simulink model "simu_v3"  (R2021a)
settings: Solver=VariableStepAuto  StartTime=0.0  StopTime=200  RelTol=1e-3
model workspace: external: MATLAB File G:\My Drive\0. PUCP\Cursos\2020.2\IEE243 - Sistemas de Control\Tarea Academica\Simulacion Robot Movil\cad files\RobotMovil_DataFile.m (data not in the file)
values from neighbouring files (symbols this model uses):
  xPla = 3    [RobotMovil_DataFile.m]
  yPla = 3    [RobotMovil_DataFile.m]
  zPla = 0.001    [RobotMovil_DataFile.m]
undefined symbols (not defined in the file or in its folder): smiData, X, Y, Z
libraries: sm_lib x211, nesl_utility x6, simulink x3, fl_lib x3
(part 5 of 5)

== system simu_v3/MODELO CINEMÁTICO ROBOT MOVIL1/RobotMovilBase_2_RIGID/shield_rb_1_RIGID/shield_rb_step_1_RIGID/tc_3528_step_1_RIGID ==
  ReferenceFrame : sm_lib/Frames and Transforms/Reference Frame
  Solid : sm_lib/Body Elements/File Solid  ExtGeomFileName=tc_3528.step_Default_sldprt.STEP  UnitType=FromFile  ExtGeomFileUnits=m  StepReaderType=HEX  ExportConvexHullGeometry=off  InertiaType=Custom  Mass=smiData.Solid(7).mass  MassUnits=kg  CenterOfMass=smiData.Solid(7).CoM  CenterOfMassUnits=mm  MomentsOfInertia=smiData.Solid(7).MoI  MomentsOfInertiaUnits=kg*mm^2  ProductsOfInertia=smiData.Solid(7).PoI  ProductsOfInertiaUnits=kg*mm^2  BasedOnType=DensityFromFile  Density=1000  DensityUnits=kg/m^3  DoExposeReferenceFrame=on  SerializedFrames=<Frames/>  GraphicType=FromGeometry  MarkerShape=Sphere  MarkerSize=10  GraphicVisPropType=SimpleVisualProperties  GraphicDiffuseColor=smiData.Solid(7).color  GraphicSpecularColor=[0.5 0.5 0.5 1.0]  GraphicAmbientColor=[0.15 0.15 0.15 1.0]  GraphicEmissiveColor=[0.0 0.0 0.0 1.0]  GraphicShininess=75  GraphicOpacity=smiData.Solid(7).opacity
  F : PMIOPort  Side=Left
  connections:
  Solid/RConn1 -- ReferenceFrame/RConn1 -- F/RConn1

== matlab function simu_v3/Controlador de Seguimiento de Trayectoria1 ==
  data: xd input; yd input; xdp input; w_ref output; ydp input; x input; y input; u_ref output; phi input
function [w_ref, u_ref] = fcn(xd,yd,xdp,ydp,x,y,phi)

a = 0.147/2;
K1 = 16;%Tes=0.25 seg
K2 = 16;%Tes=0.25 seg
%phi en radianes
xa = x + a*cos(phi);
ya = y + a*sin(phi);
%definimos la matriz M
detM=a;
Minv_11 = a*cos(phi)/detM;
Minv_12 = a*sin(phi)/detM;
Minv_21 = -sin(phi)/detM;
Minv_22 = cos(phi)/detM;
%
av1 = xdp + K1*(xd-xa);
av2 = ydp + K2*(yd-ya);
%
u_ref = Minv_11*av1 + Minv_12*av2;
w_ref = Minv_21*av1 + Minv_22*av2;%está radianes

== matlab function simu_v3/Trayectoria circular ==
  data: u input; xd output; yd output; xdp output; ydp output
function [xd,yd,xdp,ydp] = fcn(u)
persistent t
if isempty(t)
    t=0;
   
end
R=5;
xd=R*cos(2*pi*0.1*t);
yd=R*sin(2*pi*0.1*t);
xdp=-R*sin(2*pi*0.1*t)*2*pi*0.1;
ydp=R*sin(2*pi*0.1*t)*2*pi*0.1;
% xd=4.5*cosd(0)*t;
% yd=4.5*sind(0)*t;
% xdp=4.5*cosd(0);
%ydp=4.5*sind(0);
t = t + 0.25;

== matlab function simu_v3/MATLAB Function1 ==
  data: x input; xa output; y input; phi input; ya output
function [xa,ya] = fcn(x,y,phi)

a = 0.147/2;

xa = x + a*cos(phi);
ya = y + a*sin(phi);

== matlab function simu_v3/Trayectoria1 ==
  data: u input; xd output; yd output; xdp output; ydp output
function [xd,yd,xdp,ydp] = fcn(u)
persistent t
persistent xo
persistent yo
persistent camino_1
persistent camino_2
persistent camino_3
persistent camino_4
persistent camino_5
persistent camino_6
persistent camino_7
persistent camino_8
persistent camino_9
persistent camino_10
persistent camino_11
persistent camino_12
persistent camino_13
persistent camino_14
persistent camino_15
persistent camino_16
persistent camino_17
persistent camino_18
persistent camino_19
persistent camino_20

if isempty(t)
    t=0;
    xo=0;
    yo=0;
    camino_1=true;
    camino_2=true;
    camino_3=true;
    camino_4=true;
    camino_5=true;
    camino_6=true;
    camino_7=true;
    camino_8=true;
    camino_9=true;
    camino_10=true;
    camino_11=true;
    camino_12=true;
    camino_13=true;
    camino_14=true;
    camino_15=true;
    camino_16=true;
    camino_17=true;
    camino_18=true;
    camino_19=true;
    camino_20=true;
end
if camino_1
    xd=0.045*cosd(15)*t;
    yd=0.045*sind(15)*t;
    xdp=0.45*cosd(15);
    ydp=0.45*sind(15);
    d_recorrida=0.045*t; %velocidad*tiempo
    t = t + 34.6/3;
    if d_recorrida>=5.190%definir distancia
        %añadir el centro
        camino_1=false;
        xo=xd-3*sind(15);
        yo=yd+3*cond(15);
        t=0;
    end
elseif camino_2
    xd=xo+3*cosd(-75+t);
    yd=yo+3*sind(-75+t);
    %derivada
    xdp=3*-sind(-75+t);
    ydp=3*cosd(-75+t);
    if t>=42
        camino_2=false;
        xo=xd;
        yo=yd;
        t=0;
    else
        t = t + 4.2;     
    end
elseif camino_3
    xd=xo+0.045*cosd(57)*t;
    yd=yo+0.045*sind(57)*t;
    xdp=0.045*cosd(57);
    ydp=0.045*sind(57);
    d_recorrida=0.045*t; %velocidad*tiempo
    t = t + 34.6/3;
    if d_recorrida>=5.19
        %añadir el centro
        camino_3=false;
        xo=xd+cosd(33);
        yo=yd-sind(33);
        t=0;
    end    
elseif camino_4
    xd=xo+cosd(148-t);
    yd=yo+sind(148-t);
    xdp=sind(148-t);
    ydp=-cosd(148-t);
    if t>=114
        camino_4=false;
        xo=xd;
        yo=yd;
        t=0;
    else
        t = t + 11.4;     
    end
elseif camino_5
    xd=xo+0.045*cosd(-57)*t;
    yd=yo+0.045*sind(-57)*t;
    xdp=0.045*cosd(-57);
    ydp=0.045*sind(-57);
    d_recorrida=0.045*t; %velocidad*tiempo
    t = t + 34.6/3;
    if d_recorrida>=5.19
        %añadir el centro
        camino_5=false;
        xo=xd+3*cosd(33);
        yo=yd+3*sind(33);
        t=0;
    end  
elseif camino_6
    xd=xo+3*cosd(213+t);
    yd=yo+3*sind(213+t);
    %derivada?
    xdp=3*-sind(213+t);
    ydp=3*cosd(213+t);
    if t>=42
        camino_6=false;
        xo=xd;
        yo=yd;
        t=0;
    else
        t = t + 4.2;     
    end
elseif camino_7
    xd=xo+0.045*cosd(-15)*t;
    yd=yo+0.045*sind(-15)*t;
    xdp=0.045*cosd(-15);
    ydp=0.045*sind(-15);
    d_recorrida=0.045*t; %velocidad*tiempo
    t = t + 34.6/3;
    if d_recorrida>=5.19
        %añadir el centro
        camino_7=false;
        xo=xd-sind(15);
        yo=yd-cosd(15);
        t=0;
    end    
elseif camino_8
    xd=xo+cosd(75-t);
    yd=yo+sind(75-t);
    %derivada?
    xdp=sind(75-t);
    ydp=-cosd(75-t);
    if t>=114
        camino_8=false;
        xo=xd;
        yo=yd;
        t=0;
    else
        t = t + 11.4;     
    end
elseif camino_9
    xd=xo+0.045*cosd(-129)*t;
    yd=yo+0.045*sind(-129)*t;
    xdp=0.045*cosd(-129);
    ydp=0.045*sind(-129);
    d_recorrida=0.045*t; %velocidad*tiempo
    t = t + 34.6/3;
    if d_recorrida>=5.19
        %añadir el centro
        camino_9=false;
        xo=xd+3*cosd(39);
        yo=yd-3*sind(39);
        t=0;
    end
elseif camino_10
    xd=xo+3*cosd(144+t);
    yd=yo+3*sind(144+t);
    xdp=3*-sind(144+t);
    ydp=3*cosd(144+t);
    if t>=39
        camino_10=false;
        xo=xd;
        yo=yd;
        t=0;
    else
        t = t + 3.9;     
    end 
elseif camino_11 
    xd=xo;
    yd=yo-0.045*t;
    xdp=0;
    ydp=-0.045;
    d_recorrida=0.045*t; %velocidad*tiempo
    t = t + 34.6/3;
    if d_recorrida>=5.19
        %añadir el centro
        camino_11=false;
        xo=xd-1;
        yo=yd;
        t=0;
    end
elseif camino_12
    xd=xo+cosd(-t);
    yd=yo+sind(-t);
    xdp=sind(-t);
    ydp=-cosd(-t);
    if t>=108
        camino_12=false;
        xo=xd;
        yo=yd;
        t=0;
    else
        t = t + 10.8;     
    end
elseif camino_13
    xd=xo+0.045*cosd(162)*t;
    yd=yo+0.045*sind(162)*t;
    xdp=0.045*cosd(162);
    ydp=0.045*sind(162);
    d_recorrida=0.045*t; %velocidad*tiempo
    t = t + 34.6/3;
    if d_recorrida>=5.19
        %añadir el centro
        camino_13=false;
        xo=xd-3*sind(18);
        yo=yd-3*cosd(18);
        t=0;
    end
elseif camino_14
    xd=xo+3*cosd(72+t);
    yd=yo+3*sind(72+t);
    xdp=-3*sind(72+t);
    ydp=3*cosd(72+t);
    if t>=36
        camino_14=false;
        xo=xd;
        yo=yd;
        t=0;
    else
        t = t + 3.6;     
    end
elseif camino_15
    xd=xo+0.045*cosd(198)*t;
    yd=yo+0.045*sind(198)*t;
    xdp=0.045*cosd(198);
    ydp=0.045*sind(198);
    d_recorrida=0.045*t; %velocidad*tiempo
    t = t + 34.6/3;
    if d_recorrida>=5.19
        %añadir el centro
        camino_15=false;
        xo=xd-sind(18);
        yo=yd+cosd(18);
        t=0;
    end
elseif camino_16
    xd=xo+cosd(-72-t);
    yd=yo+sind(-72-t);
    xdp=sind(-72-t);
    ydp=-cosd(-72-t);
    if t>=108
        camino_16=false;
        xo=xd;
        yo=yd;
        t=0;
    else
        t = t + 10.8;     
    end
elseif camino_17
    xd=xo;
    yd=yo+0.045*t;
    xdp=0;
    ydp=0.045;
    d_recorrida=0.045*t; %velocidad*tiempo
    t = t + 34.6/3;
    if d_recorrida>=5.19
        %añadir el centro
        camino_17=false;
        xo=xd-3;
        yo=yd;
        t=0;
    end
elseif camino_18
    xd=xo+3*cosd(t);
    yd=yo+3*sind(t);
    xdp=3*sind(t);
    ydp=-3*cosd(t);
    if t>=39
        camino_18=false;
        xo=xd;
        yo=yd;
        t=0;
    else
        t = t + 3.9;     
    end
elseif camino_19
    xd=xo+0.045*cosd(129)*t;
    yd=yo+0.045*sind(129)*t;
    xdp=0.045*cosd(129);
    ydp=0.045*sind(129);
    d_recorrida=0.045*t; %velocidad*tiempo
    t = t + 34.6/3;
    if d_recorrida>=5.19
        %añadir el centro
        camino_19=false;
        xo=xd+cosd(39);
        yo=yd+sind(39);
        t=0;
    end
elseif camino_20
    xd=xo+cosd(219-t);
    yd=yo+sind(219-t);
    xdp=sind(219-t);
    ydp=-cosd(219-t);
    if t>=114
        camino_20=false;
        xo=xd;
        yo=yd;
        t=0;
    else
        t = t + 11.4;     
    end
else
    xd=0;
    yd=0;
    xdp=0;
    ydp=0;
    t=0;
    xo=0;
    yo=0;
    camino_1=true;
    camino_2=true;
    camino_3=true;
    camino_4=true;
    camino_5=true;
    camino_6=true;
    camino_7=true;
    camino_8=true;
    camino_9=true;
    camino_10=true;
    camino_11=true;
    camino_12=true;
    camino_13=true;
    camino_14=true;
    camino_15=true;
    camino_16=true;
    camino_17=true;
    camino_18=true;
    camino_19=true;
    camino_20=true;
end
%para reducir el tamaño de la estrella
xd=xd/10;
yd=yd/10;
xdp=xdp/10;
ydp=ydp/10;

== matlab function simu_v3/Control velocidad/Control Derecho/PI2 ==
  data: e input; u output
function u = fcn(e)

persistent ud_1
persistent ed_1
if isempty(ud_1)
    ud_1=0;
    ed_1=0;
end
Ts=0.01;
Kp = 0.0208;
Ki = 0.1248;
u=ud_1+(2*Kp+Ki*Ts)/2*e+(Ki*Ts-2*Kp)/2*ed_1;
ed_1=e;
ud_1=u;

== matlab function simu_v3/Control velocidad/Control izquierdo/PI2 ==
  data: e input; u output
function u = fcn(e)

persistent ui_1
persistent ei_1
if isempty(ui_1)
    ui_1=0;
    ei_1=0;
end
Ts=0.006;
Kp=0.020056241439231;
Ki=0.441237311663075;
u=ui_1+(2*Kp+Ki*Ts)/2*e+(Ki*Ts-2*Kp)/2*ei_1;
ei_1=e;
ui_1=u;
